simulink model "A1_PaceMaker"  (R2022a)
settings: Solver=FixedStepAuto  StartTime=0.0  StopTime=10.0  FixedStep=1e-3  RelTol=1e-3  EnableMultiTasking=on
undefined symbols (not defined in the file): D0, D1, D10, D11, D12, D13, D2, D3, D4, D5, D6, D7, D8, D9, PTA0, PTA1, PTA2, PTB23, PTB9, PTC16, PTC17, PTC2, PTC3, PTC4, PTD0, PTD1, PTD2, PTD3
libraries: frdmk64flib x14
settings Model: ExtModeTrigDuration=5  Creator=ramu7  LastModifiedBy=scoob
settings OptimizationCC: EnhancedBackFolding=on  PassReuseOutputArgsAs=Individual arguments  ZeroExternalMemoryAtStartup=off  ZeroInternalMemoryAtStartup=off  MaxStackSize=64  OptimizeBlockOrder=speed  DifferentSizesBufferReuse=on  OptimizationCustomize=off  EfficientTunableParamExpr=on
settings DebuggingCC: ParameterTunabilityLossMsg=error
settings HardwareCC: ProdBitPerPointer=32  ProdBitPerSizeT=32  ProdBitPerPtrDiffT=32  ProdLargestAtomicInteger=Long  ProdLargestAtomicFloat=Double  ProdWordSize=32  ProdHWDeviceType=ARM Compatible->ARM Cortex
settings SFSimCC: MATLABDynamicMemAlloc=off
settings RTWCC: SystemTargetFile=ert.tlc  HardwareBoard=NXP FRDM-K64F  TLCOptions="-aInlineSetEventsForThisBaseRateFcn=TLC_FALSE -aSuppressMultiTaskScheduler=TLC_FALSE  -aRateBasedStepFcn=0"  TemplateMakefile=ert_default_tmf  Toolchain=GNU Tools for ARM Embedded Processors
settings CodeAppCC: ForceParamTrailComments=on  IgnoreCustomStorageClasses=off  OperatorAnnotations=on  SimulinkDataObjDesc=on  SFDataObjDesc=on  InsertBlockDesc=on
settings ERTTargetCC: ExtModeTransport=4  ExtModeMexFile=sendToCommService

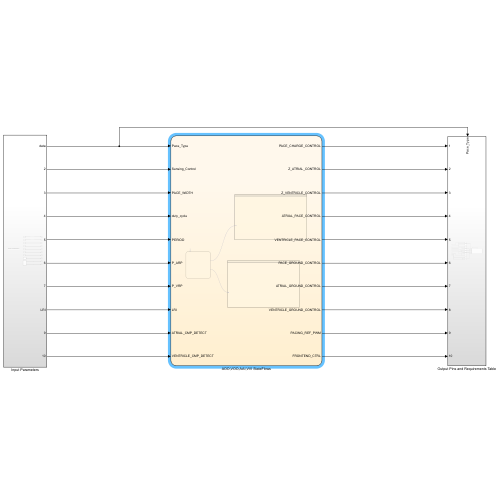
[thumbnail: Simulink's stored preview of the top-level diagram]
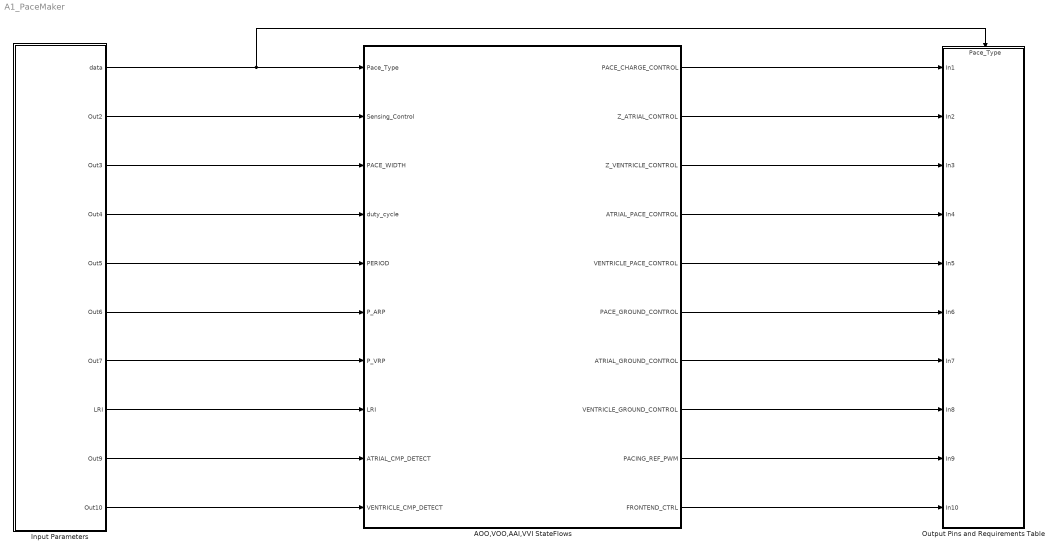
== system A1_PaceMaker ==
  AOO,VOO,AAI,VVI StateFlows : Stateflow chart  TreatAsAtomicUnit=on
      settings: PortSchema="{\"entries\":[{\"content\":{\"sides\":[{\"content\":{\"connectorIds\":[\"In2\",\"In10\",\"In7\",\"In1\",\"In3\",\"In9\",\"In8\",\"In6\",\"In4\",\"In5\"]},\"type\":\"ConnectorPlacement.EquallySpacedRectSide\",\"uuid\":\"9770646f-499d-4715-b3e0-54ec63e9a743\"},{\"content\":{\"connectorIds\":[\"Out1\",\"Out2\",\"Out3\",\"Out4\",\"Out5\",\"Out6\",\"Out7\",\"Out8\",\"Out9\",\"Out10\"],\"side\":\"RIGHT\"},\"type\":\"ConnectorPlacement.EquallySpacedRectSide\",\"uuid\":\"05a40026-c63e-4ef0-b71d-820a20f884f3\"},{\"content\":{\"connectorIds\":[],\"side\":\"TOP\"},\"type\":\"ConnectorPlacement.EquallySpacedRectSide\",\"uuid\":\"87d8712c-6353-4ad8-9661-243ca412d6bb\"}]},\"type\":\"ConnectorPlacement.EquallySpacedConnector\",\"uuid\":\"8262e7ac-98b5-44bf-add5-1ad3a0c707a1\"}],\"packageUris\":[\"http://schema.mathworks.com/mf0/Connector/R2020b\"],\"version\":\"1.0\"}"
  Input Parameters : Subsystem
  Output Pins and Requirements Table : Subsystem
      settings: PortSchema="{\"entries\":[{\"content\":{\"sides\":[{\"content\":{\"connectorIds\":[\"In1\",\"In2\",\"In3\",\"In4\",\"In5\",\"In6\",\"In7\",\"In8\",\"In9\",\"In10\"]},\"type\":\"ConnectorPlacement.EquallySpacedRectSide\",\"uuid\":\"40db26f6-8e31-4589-a315-6eea3b6d58f2\"},{\"content\":{\"connectorIds\":[],\"side\":\"RIGHT\"},\"type\":\"ConnectorPlacement.EquallySpacedRectSide\",\"uuid\":\"a6caef76-430e-44a7-94fa-313885a27199\"},{\"content\":{\"connectorIds\":[\"In11\"],\"side\":\"TOP\"},\"type\":\"ConnectorPlacement.EquallySpacedRectSide\",\"uuid\":\"9adbd5f8-a295-4590-a052-0a7aa200e456\"}]},\"type\":\"ConnectorPlacement.EquallySpacedConnector\",\"uuid\":\"6d560563-586d-4d61-8602-6a07324ae70c\"}],\"packageUris\":[\"http://schema.mathworks.com/mf0/Connector/R2020b\"],\"version\":\"1.0\"}"
  wires:
  AOO,VOO,AAI,VVI StateFlows/10(FRONTEND_CTRL) -> Output Pins and Requirements Table/10(In10)
  Input Parameters/8(LRI) -> AOO,VOO,AAI,VVI StateFlows/6(LRI)
  AOO,VOO,AAI,VVI StateFlows/6(PACE_GROUND_CONTROL) -> Output Pins and Requirements Table/6(In6)
  AOO,VOO,AAI,VVI StateFlows/2(Z_ATRIAL_CONTROL) -> Output Pins and Requirements Table/2(In2)
  AOO,VOO,AAI,VVI StateFlows/3(Z_VENTRICLE_CONTROL) -> Output Pins and Requirements Table/3(In3)
  AOO,VOO,AAI,VVI StateFlows/1(PACE_CHARGE_CONTROL) -> Output Pins and Requirements Table/1(In1)
  AOO,VOO,AAI,VVI StateFlows/4(ATRIAL_PACE_CONTROL) -> Output Pins and Requirements Table/4(In4)
  Input Parameters/3(Out3) -> AOO,VOO,AAI,VVI StateFlows/7(PACE_WIDTH)
  AOO,VOO,AAI,VVI StateFlows/9(PACING_REF_PWM) -> Output Pins and Requirements Table/9(In9)
  Input Parameters/2(Out2) -> AOO,VOO,AAI,VVI StateFlows/10(Sensing_Control)
  Input Parameters/5(Out5) -> AOO,VOO,AAI,VVI StateFlows/3(PERIOD)
  AOO,VOO,AAI,VVI StateFlows/7(ATRIAL_GROUND_CONTROL) -> Output Pins and Requirements Table/7(In7)
  Input Parameters/9(Out9) -> AOO,VOO,AAI,VVI StateFlows/4(ATRIAL_CMP_DETECT)
  Input Parameters/4(Out4) -> AOO,VOO,AAI,VVI StateFlows/1(duty_cycle)
  AOO,VOO,AAI,VVI StateFlows/5(VENTRICLE_PACE_CONTROL) -> Output Pins and Requirements Table/5(In5)
  Input Parameters/7(Out7) -> AOO,VOO,AAI,VVI StateFlows/8(P_VRP)
  Input Parameters/10(Out10) -> AOO,VOO,AAI,VVI StateFlows/5(VENTRICLE_CMP_DETECT)
  AOO,VOO,AAI,VVI StateFlows/8(VENTRICLE_GROUND_CONTROL) -> Output Pins and Requirements Table/8(In8)
  Input Parameters/6(Out6) -> AOO,VOO,AAI,VVI StateFlows/9(P_ARP)
  Input Parameters/1(data) -> Output Pins and Requirements Table/11(Pace_Type), AOO,VOO,AAI,VVI StateFlows/2(Pace_Type)

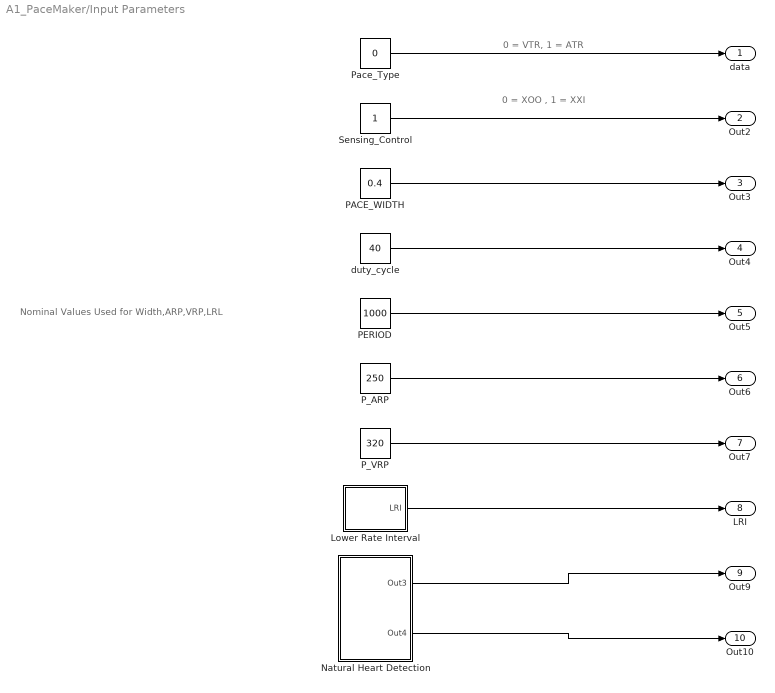
== system A1_PaceMaker/Input Parameters ==
  note: Nominal Values Used for Width,ARP,VRP,LRL
  note: 0 = XOO , 1 = XXI
  note: 0 = VTR, 1 = ATR
  Lower Rate Interval : Subsystem
  Natural Heart Detection : Subsystem
  PACE_WIDTH : Constant  Value=0.4
  PERIOD : Constant  Value=1000
  P_ARP : Constant  Value=250
  P_VRP : Constant  Value=320
  Pace_Type : Constant  Value=0  OutDataTypeStr=boolean
  Sensing_Control : Constant  OutDataTypeStr=boolean
  duty_cycle : Constant  Value=40  OutDataTypeStr=double
  data : Outport
  Out2 : Outport  Port=2
  Out3 : Outport  Port=3
  Out4 : Outport  Port=4
  Out5 : Outport  Port=5
  Out6 : Outport  Port=6
  Out7 : Outport  Port=7
  LRI : Outport  Port=8
  Out9 : Outport  Port=9
  Out10 : Outport  Port=10
  wires:
  Lower Rate Interval/1(LRI) -> LRI/1
  PERIOD/1 -> Out5/1
  P_VRP/1 -> Out7/1
  duty_cycle/1 -> Out4/1
  Sensing_Control/1 -> Out2/1
  PACE_WIDTH/1 -> Out3/1
  Natural Heart Detection/2(Out4) -> Out10/1
  P_ARP/1 -> Out6/1
  Pace_Type/1 -> data/1
  Natural Heart Detection/1(Out3) -> Out9/1

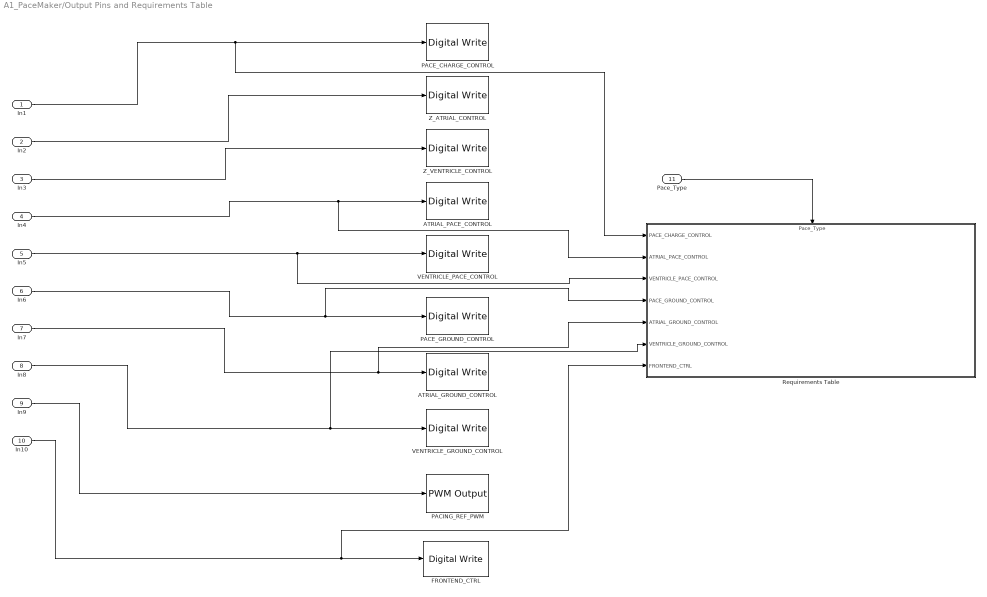
== system A1_PaceMaker/Output Pins and Requirements Table ==
  In1 : Inport
  In2 : Inport  Port=2
  In3 : Inport  Port=3
  In4 : Inport  Port=4
  In5 : Inport  Port=5
  In6 : Inport  Port=6
  In7 : Inport  Port=7
  In8 : Inport  Port=8
  In9 : Inport  Port=9
  In10 : Inport  Port=10
  Pace_Type : Inport  Port=11
  ATRIAL_GROUND_CONTROL : frdmk64flib/Digital Write  Whichpin=PTD2 (D11)
  ATRIAL_PACE_CONTROL : frdmk64flib/Digital Write  Whichpin=PTA0 (D8)
  FRONTEND_CTRL : frdmk64flib/Digital Write  Whichpin=PTD1 (D13)
  PACE_CHARGE_CONTROL : frdmk64flib/Digital Write  Whichpin=PTB9 (D2)
  PACE_GROUND_CONTROL : frdmk64flib/Digital Write  Whichpin=PTD0 (D10)
  PACING_REF_PWM : frdmk64flib/PWM Output  Whichpin=PTA2 (D5)  InitialFrequency=2000  InitialDutyCycle=40
  Requirements Table : Subsystem
      settings: PortSchema="{\"entries\":[{\"content\":{\"sides\":[{\"content\":{\"connectorIds\":[\"In1\",\"In2\",\"In3\",\"In4\",\"In5\",\"In6\",\"In7\"]},\"type\":\"ConnectorPlacement.EquallySpacedRectSide\",\"uuid\":\"46327938-4478-40d2-aac6-72547228615e\"},{\"content\":{\"connectorIds\":[],\"side\":\"RIGHT\"},\"type\":\"ConnectorPlacement.EquallySpacedRectSide\",\"uuid\":\"a4c12f67-beb4-4537-be9d-262931108289\"},{\"content\":{\"connectorIds\":[\"In8\"],\"side\":\"TOP\"},\"type\":\"ConnectorPlacement.EquallySpacedRectSide\",\"uuid\":\"a653f2ff-3266-45dd-85b5-df796fc313fd\"}]},\"type\":\"ConnectorPlacement.EquallySpacedConnector\",\"uuid\":\"ede91063-bb98-4867-a1df-25b64c24a60e\"}],\"packageUris\":[\"http://schema.mathworks.com/mf0/Connector/R2020b\"],\"version\":\"1.0\"}"
  VENTRICLE_GROUND_CONTROL : frdmk64flib/Digital Write  Whichpin=PTD3 (D12)
  VENTRICLE_PACE_CONTROL : frdmk64flib/Digital Write  Whichpin=PTC4 (D9)
  Z_ATRIAL_CONTROL : frdmk64flib/Digital Write  Whichpin=PTB23 (D4)
  Z_VENTRICLE_CONTROL : frdmk64flib/Digital Write  Whichpin=PTC3 (D7)
  wires:
  In2/1 -> Z_ATRIAL_CONTROL/1
  In9/1 -> PACING_REF_PWM/1
  In5/1 -> Requirements Table/3(VENTRICLE_PACE_CONTROL), VENTRICLE_PACE_CONTROL/1
  In7/1 -> Requirements Table/5(ATRIAL_GROUND_CONTROL), ATRIAL_GROUND_CONTROL/1
  In4/1 -> Requirements Table/2(ATRIAL_PACE_CONTROL), ATRIAL_PACE_CONTROL/1
  In8/1 -> Requirements Table/6(VENTRICLE_GROUND_CONTROL), VENTRICLE_GROUND_CONTROL/1
  In6/1 -> Requirements Table/4(PACE_GROUND_CONTROL), PACE_GROUND_CONTROL/1
  In1/1 -> Requirements Table/1(PACE_CHARGE_CONTROL), PACE_CHARGE_CONTROL/1
  In3/1 -> Z_VENTRICLE_CONTROL/1
  In10/1 -> Requirements Table/7(FRONTEND_CTRL), FRONTEND_CTRL/1
  Pace_Type/1 -> Requirements Table/8(Pace_Type)

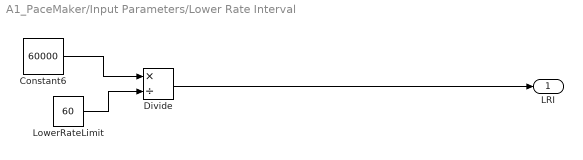
== system A1_PaceMaker/Input Parameters/Lower Rate Interval ==
  Constant6 : Constant  Value=60000
  Divide : Product  Inputs=*/
  LowerRateLimit : Constant  Value=60
  LRI : Outport
  wires:
  Constant6/1 -> Divide/1
  LowerRateLimit/1 -> Divide/2
  Divide/1 -> LRI/1

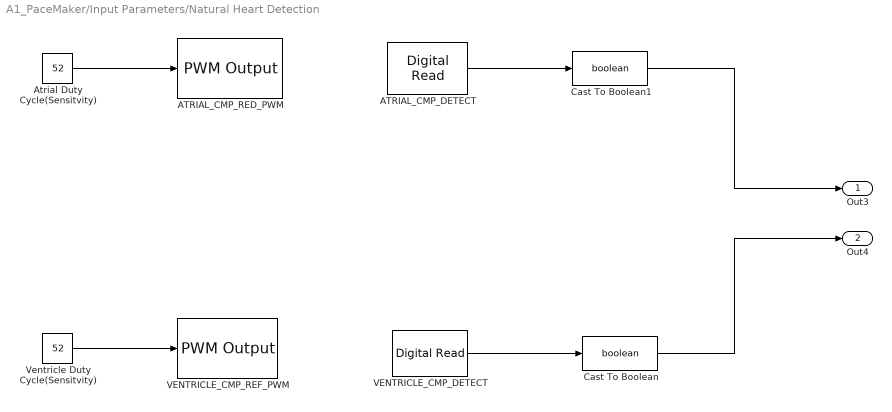
== system A1_PaceMaker/Input Parameters/Natural Heart Detection ==
  ATRIAL_CMP_DETECT : frdmk64flib/Digital Read  Whichpin=PTC16 (D0)  SampleTime=-1
  ATRIAL_CMP_RED_PWM : frdmk64flib/PWM Output  Whichpin=PTC2 (D6)  InitialFrequency=2000  InitialDutyCycle=51
  Atrial Duty Cycle(Sensitvity) : Constant  Value=52
  Cast To Boolean : DataTypeConversion  OutDataTypeStr=boolean  SaturateOnIntegerOverflow=off  RndMeth=Floor
  Cast To Boolean1 : DataTypeConversion  OutDataTypeStr=boolean  SaturateOnIntegerOverflow=off  RndMeth=Floor
  VENTRICLE_CMP_DETECT : frdmk64flib/Digital Read  Whichpin=PTC17 (D1)  SampleTime=-1
  VENTRICLE_CMP_REF_PWM : frdmk64flib/PWM Output  Whichpin=PTA1 (D3)  InitialFrequency=2000  InitialDutyCycle=60
  Ventricle Duty Cycle(Sensitvity) : Constant  Value=52
  Out3 : Outport
  Out4 : Outport  Port=2
  wires:
  Ventricle Duty Cycle(Sensitvity)/1 -> VENTRICLE_CMP_REF_PWM/1
  Atrial Duty Cycle(Sensitvity)/1 -> ATRIAL_CMP_RED_PWM/1
  VENTRICLE_CMP_DETECT/1 -> Cast To Boolean/1
  ATRIAL_CMP_DETECT/1 -> Cast To Boolean1/1
  Cast To Boolean1/1 -> Out3/1
  Cast To Boolean/1 -> Out4/1

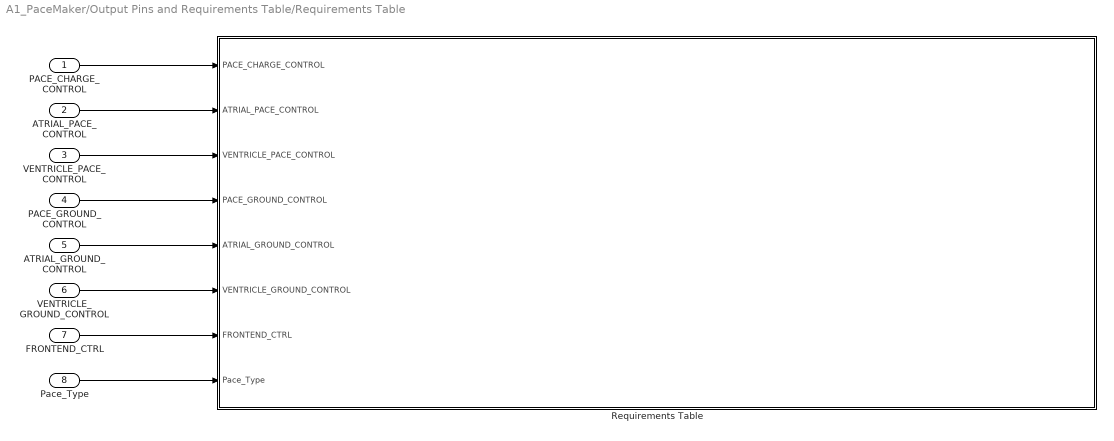
== system A1_PaceMaker/Output Pins and Requirements Table/Requirements Table ==
  PACE_CHARGE_CONTROL : Inport
  ATRIAL_PACE_CONTROL : Inport  Port=2
  VENTRICLE_PACE_CONTROL : Inport  Port=3
  PACE_GROUND_CONTROL : Inport  Port=4
  ATRIAL_GROUND_CONTROL : Inport  Port=5
  VENTRICLE_GROUND_CONTROL : Inport  Port=6
  FRONTEND_CTRL : Inport  Port=7
  Pace_Type : Inport  Port=8
  Requirements Table : Requirements Table  TreatAsAtomicUnit=on
  wires:
  PACE_CHARGE_CONTROL/1 -> Requirements Table/1(PACE_CHARGE_CONTROL)
  ATRIAL_PACE_CONTROL/1 -> Requirements Table/2(ATRIAL_PACE_CONTROL)
  VENTRICLE_PACE_CONTROL/1 -> Requirements Table/3(VENTRICLE_PACE_CONTROL)
  PACE_GROUND_CONTROL/1 -> Requirements Table/4(PACE_GROUND_CONTROL)
  ATRIAL_GROUND_CONTROL/1 -> Requirements Table/5(ATRIAL_GROUND_CONTROL)
  VENTRICLE_GROUND_CONTROL/1 -> Requirements Table/6(VENTRICLE_GROUND_CONTROL)
  FRONTEND_CTRL/1 -> Requirements Table/7(FRONTEND_CTRL)
  Pace_Type/1 -> Requirements Table/8(Pace_Type)

== stateflow chart A1_PaceMaker/AOO,VOO,AAI,VVI StateFlows ==
  state VENTRICLE MODES (VOO and VVI) [group]
    state SENSE_Ventricle
    note: Heartbeat not found after the LRI period, pace the heart
    note: Heartbeat found, reset LRI
    state PACE_Charge_Ventricle
      entry:
      PACE_CHARGE_CONTROL = true
      VENTRICLE_PACE_CONTROL = false
      VENTRICLE_GROUND_CONTROL=true
      ATRIAL_PACE_CONTROL =false
      ATRIAL_GROUND_CONTROL = false
    state PACE_Discharge_Ventricle
      entry:
      PACE_CHARGE_CONTROL = false
      VENTRICLE_PACE_CONTROL = true
      VENTRICLE_GROUND_CONTROL= false
    SENSE_Ventricle -> PACE_Discharge_Ventricle [order 1] : after(LRI - P_VRP,msec) [VENTRICLE_CMP_DETECT == false]
    SENSE_Ventricle -> PACE_Charge_Ventricle [order 2] : [VENTRICLE_CMP_DETECT == true]
    PACE_Charge_Ventricle -> SENSE_Ventricle [order 1] : after(P_VRP,msec)[Sensing_Control == true]
    PACE_Charge_Ventricle -> PACE_Discharge_Ventricle [order 2] : after(PERIOD - PACE_WIDTH,msec)[Sensing_Control == false]
    PACE_Discharge_Ventricle -> PACE_Charge_Ventricle : after(PACE_WIDTH,msec)
  state init_state
    entry:
    PACING_REF_PWM = duty_cycle
    Z_ATRIAL_CONTROL = false
    Z_VENTRICLE_CONTROL = false
    PACE_GROUND_CONTROL = true
    FRONTEND_CTRL = true
  state ATRIAL MODES (AOO and AAI) [group]
    state SENSE_Atrial
    note: Heartbeat not found after the LRI period, pace the heart
    note: Heartbeat found, reset LRI
    state PACE_Charge_Atrial
      entry:
      PACE_CHARGE_CONTROL = true
      VENTRICLE_PACE_CONTROL = false
      VENTRICLE_GROUND_CONTROL=false
      ATRIAL_PACE_CONTROL =false
      ATRIAL_GROUND_CONTROL = true
    state PACE_Discharge_Atrial
      entry:
      PACE_CHARGE_CONTROL = false
      ATRIAL_PACE_CONTROL = true
      ATRIAL_GROUND_CONTROL = false
    SENSE_Atrial -> PACE_Discharge_Atrial [order 1] : after(LRI - P_ARP - PACE_WIDTH,msec) [ATRIAL_CMP_DETECT == false]
    SENSE_Atrial -> PACE_Charge_Atrial [order 2] : [ATRIAL_CMP_DETECT == true]
    PACE_Charge_Atrial -> SENSE_Atrial [order 1] : after(P_ARP,msec) [Sensing_Control == true]
    PACE_Charge_Atrial -> PACE_Discharge_Atrial [order 2] : after(PERIOD - PACE_WIDTH,msec)[Sensing_Control == false]
    PACE_Discharge_Atrial -> PACE_Charge_Atrial : after(PACE_WIDTH,msec)
  init_state -> PACE_Charge_Ventricle [order 2] : [Pace_Type == 0]
  (default) -> init_state
  init_state -> PACE_Charge_Atrial [order 1] : [Pace_Type == 1]
  data: PACE_CHARGE_CONTROL output; Z_ATRIAL_CONTROL output; Z_VENTRICLE_CONTROL output; ATRIAL_PACE_CONTROL output; VENTRICLE_PACE_CONTROL output; PACE_GROUND_CONTROL output; ATRIAL_GROUND_CONTROL output; VENTRICLE_GROUND_CONTROL output; PACING_REF_PWM output; duty_cycle input; Pace_Type input boolean; PERIOD input double; ATRIAL_CMP_DETECT input boolean; VENTRICLE_CMP_DETECT input boolean; LRI input double; PACE_WIDTH input double; P_VRP input double; P_ARP input double; Sensing_Control input boolean; FRONTEND_CTRL output boolean

== stateflow chart A1_PaceMaker/Output Pins and Requirements Table/Requirements Table/Requirements Table ==
  (default) -> (junction 1073754047)
  (junction 1073754047) -> (junction 1073754048) : {
      | % SF_REQ_REV_07
      | }
  (junction 1073754048) -> (junction 1073754050) : {
      | % HEADER_ASSIGNMENTS
      |
      | }
  (junction 1073754050) -> (junction 1073754052) : {
      | % START_A_4
      | }
  (junction 1073754052) -> (junction 1073754054) : {
      | }
  (junction 1073754054) -> (junction 1073754056)
  (junction 1073754056) -> (junction 1073754058) : {
      | }
  (junction 1073754058) -> (junction 1073754060) : {
      | % END_A_4
      | }
  (junction 1073754060) -> (junction 1073754062) : {
      | % START_R_1
      | }
  (junction 1073754062) -> (junction 1073754064) : {
      | }
  (junction 1073754064) -> (junction 1073754066)
  (junction 1073754066) -> (junction 1073754068) [order 1] : [(((Front End Control) == (FRONTEND_CTRL==1))) && (((Pace Ground Control) == (PACE_GROUND_CONTROL==1))) && (((Z Atrial Control) == (Z_ATRIAL_CONTROL==0))) && (((Z Ventricular Control) == (Z_VENTRICLE_CONTROL==0))) && (((Pace Type) == (Pace_Type==1)))]
  (junction 1073754066) -> (junction 1073754164) [order 2]
  (junction 1073754068) -> (junction 1073754070) : {
      | reqtable_postcondition((((PACE_CHARGE_CONTROL) == (1))) && (((VENTRICLE_PACE_CONTROL) == (0))) && (((VENTRICLE_GROUND_CONTROL) == (0))) && (((ATRIAL_PACE_CONTROL) == (0))) && (((ATRIAL_GROUND_CONTROL) == (1))), 'R:1');
      |
      |
      | }
  (junction 1073754070) -> (junction 1073754072) : {
      | }
  (junction 1073754072) -> (junction 1073754074) : {
      | % START_R_10
      | }
  (junction 1073754074) -> (junction 1073754076) : {
      | }
  (junction 1073754076) -> (junction 1073754078)
  (junction 1073754078) -> (junction 1073754080) [order 1] : [(((Pace Charge Control) == (PACE_CHARGE_CONTROL==1))) && (((Ventricle Pace Control) == (VENTRICLE_PACE_CONTROL==0))) && (((Ventricle Ground Control) == (VENTRICLE_GROUND_CONTROL==0))) && (((Atrial Pace Control) == (ATRIAL_PACE_CONTROL==0))) && (((Atrial Ground Control) == (ATRIAL_GROUND_CONTROL==1))) && (((Sensing Control) == (Sensing_Control==0)))]
  (junction 1073754078) -> (junction 1073754086) [order 2]
  (junction 1073754080) -> (junction 1073754082) : {
      | reqtable_postcondition((((PACE_CHARGE_CONTROL) == (0))) && (((ATRIAL_PACE_CONTROL) == (1))) && (((ATRIAL_GROUND_CONTROL) == (0))), 'R:1.1');
      |
      |
      | }
  (junction 1073754082) -> (junction 1073754084) : {
      | }
  (junction 1073754084) -> (junction 1073754086)
  (junction 1073754086) -> (junction 1073754088)
  (junction 1073754088) -> (junction 1073754090) : {
      | % END_R_10
      | }
  (junction 1073754090) -> (junction 1073754092) : {
      | % START_R_16
      | }
  (junction 1073754092) -> (junction 1073754094) : {
      | }
  (junction 1073754094) -> (junction 1073754096)
  (junction 1073754096) -> (junction 1073754098) [order 1] : [(((Pace Charge Control) == (PACE_CHARGE_CONTROL==0))) && (((Atrial Pace Control) == (ATRIAL_PACE_CONTROL==1))) && (((Atrial Ground Control) == (ATRIAL_GROUND_CONTROL==0)))]
  (junction 1073754096) -> (junction 1073754104) [order 2]
  (junction 1073754098) -> (junction 1073754100) : {
      | reqtable_postcondition((((PACE_CHARGE_CONTROL) == (1))) && (((VENTRICLE_PACE_CONTROL) == (0))) && (((VENTRICLE_GROUND_CONTROL) == (0))) && (((ATRIAL_PACE_CONTROL) == (0))) && (((ATRIAL_GROUND_CONTROL) == (1))), 'R:1.2');
      |
      |
      | }
  (junction 1073754100) -> (junction 1073754102) : {
      | }
  (junction 1073754102) -> (junction 1073754104)
  (junction 1073754104) -> (junction 1073754106)
  (junction 1073754106) -> (junction 1073754108) : {
      | % END_R_16
      | }
  (junction 1073754108) -> (junction 1073754110) : {
      | % START_R_19
      | }
  (junction 1073754110) -> (junction 1073754112) : {
      | }
  (junction 1073754112) -> (junction 1073754114)
  (junction 1073754114) -> (junction 1073754116) [order 1] : [(((Pace Charge Control) == (PACE_CHARGE_CONTROL==1))) && (((Ventricle Pace Control) == (VENTRICLE_PACE_CONTROL==0))) && (((Ventricle Ground Control) == (VENTRICLE_GROUND_CONTROL==0))) && (((Atrial Pace Control) == (ATRIAL_PACE_CONTROL==0))) && (((Atrial Ground Control) == (ATRIAL_GROUND_CONTROL==1))) && (((Sensing Control) == (Sensing_Control==1)))]
  (junction 1073754114) -> (junction 1073754122) [order 2]
  (junction 1073754116) -> (junction 1073754118) : {
      |
      |
      | }
  (junction 1073754118) -> (junction 1073754120) : {
      | }
  (junction 1073754120) -> (junction 1073754122)
  (junction 1073754122) -> (junction 1073754124)
  (junction 1073754124) -> (junction 1073754126) : {
      | % END_R_19
      | }
  (junction 1073754126) -> (junction 1073754128) : {
      | % START_R_28
      | }
  (junction 1073754128) -> (junction 1073754130) : {
      | }
  (junction 1073754130) -> (junction 1073754132)
  (junction 1073754132) -> (junction 1073754134) [order 1] : [(((Atrial CMP Detect) == (ATRIAL_CMP_DETECT==1)))]
  (junction 1073754132) -> (junction 1073754140) [order 2]
  (junction 1073754134) -> (junction 1073754136) : {
      | reqtable_postcondition((((PACE_CHARGE_CONTROL) == (1))) && (((VENTRICLE_PACE_CONTROL) == (0))) && (((VENTRICLE_GROUND_CONTROL) == (0))) && (((ATRIAL_PACE_CONTROL) == (0))) && (((ATRIAL_GROUND_CONTROL) == (1))), 'R:1.4');
      |
      |
      | }
  (junction 1073754136) -> (junction 1073754138) : {
      | }
  (junction 1073754138) -> (junction 1073754140)
  (junction 1073754140) -> (junction 1073754142)
  (junction 1073754142) -> (junction 1073754144) : {
      | % END_R_28
      | }
  (junction 1073754144) -> (junction 1073754146) : {
      | % START_R_31
      | }
  (junction 1073754146) -> (junction 1073754148) : {
      | }
  (junction 1073754148) -> (junction 1073754150)
  (junction 1073754150) -> (junction 1073754152) [order 1] : [(((Atrial CMP Detect) == (ATRIAL_CMP_DETECT==0)))]
  (junction 1073754150) -> (junction 1073754158) [order 2]
  (junction 1073754152) -> (junction 1073754154) : {
      | reqtable_postcondition((((PACE_CHARGE_CONTROL) == (0))) && (((ATRIAL_PACE_CONTROL) == (1))) && (((ATRIAL_GROUND_CONTROL) == (0))), 'R:1.5');
      |
      |
      | }
  (junction 1073754154) -> (junction 1073754156) : {
      | }
  (junction 1073754156) -> (junction 1073754158)
  (junction 1073754158) -> (junction 1073754160)
  (junction 1073754160) -> (junction 1073754162) : {
      | % END_R_31
      | }
  (junction 1073754162) -> (junction 1073754164)
  (junction 1073754164) -> (junction 1073754166)
  (junction 1073754166) -> (junction 1073754168) : {
      | % END_R_1
      | }
  (junction 1073754168) -> (junction 1073754170) : {
      | % START_R_7
      | }
  (junction 1073754170) -> (junction 1073754172) : {
      | }
  (junction 1073754172) -> (junction 1073754174)
  (junction 1073754174) -> (junction 1073754176) [order 1] : [(((Front End Control) == (FRONTEND_CTRL==1))) && (((Pace Ground Control) == (PACE_GROUND_CONTROL==1))) && (((Z Atrial Control) == (Z_ATRIAL_CONTROL==0))) && (((Z Ventricular Control) == (Z_VENTRICLE_CONTROL==0))) && (((Pace Type) == (Pace_Type==0)))]
  (junction 1073754174) -> (junction 1073754272) [order 2]
  (junction 1073754176) -> (junction 1073754178) : {
      | reqtable_postcondition((((PACE_CHARGE_CONTROL) == (1))) && (((VENTRICLE_PACE_CONTROL) == (0))) && (((VENTRICLE_GROUND_CONTROL) == (1))) && (((ATRIAL_PACE_CONTROL) == (0))) && (((ATRIAL_GROUND_CONTROL) == (0))), 'R:2');
      |
      |
      | }
  (junction 1073754178) -> (junction 1073754180) : {
      | }
  (junction 1073754180) -> (junction 1073754182) : {
      | % START_R_13
      | }
  (junction 1073754182) -> (junction 1073754184) : {
      | }
  (junction 1073754184) -> (junction 1073754186)
  (junction 1073754186) -> (junction 1073754188) [order 1] : [(((Pace Charge Control) == (PACE_CHARGE_CONTROL==1))) && (((Ventricle Pace Control) == (VENTRICLE_PACE_CONTROL==0))) && (((Ventricle Ground Control) == (VENTRICLE_GROUND_CONTROL==1))) && (((Atrial Pace Control) == (ATRIAL_PACE_CONTROL==0))) && (((Atrial Ground Control) == (ATRIAL_GROUND_CONTROL==0))) && (((Sensing Control) == (Sensing_Control==0)))]
  (junction 1073754186) -> (junction 1073754194) [order 2]
  (junction 1073754188) -> (junction 1073754190) : {
      | reqtable_postcondition((((PACE_CHARGE_CONTROL) == (0))) && (((VENTRICLE_PACE_CONTROL) == (1))) && (((VENTRICLE_GROUND_CONTROL) == (0))), 'R:2.1');
      |
      |
      | }
  (junction 1073754190) -> (junction 1073754192) : {
      | }
  (junction 1073754192) -> (junction 1073754194)
  (junction 1073754194) -> (junction 1073754196)
  (junction 1073754196) -> (junction 1073754198) : {
      | % END_R_13
      | }
  (junction 1073754198) -> (junction 1073754200) : {
      | % START_R_22
      | }
  (junction 1073754200) -> (junction 1073754202) : {
      | }
  (junction 1073754202) -> (junction 1073754204)
  (junction 1073754204) -> (junction 1073754206) [order 1] : [(((Pace Charge Control) == (PACE_CHARGE_CONTROL==0))) && (((Ventricle Pace Control) == (VENTRICLE_PACE_CONTROL==1))) && (((Ventricle Ground Control) == (VENTRICLE_GROUND_CONTROL==0)))]
  (junction 1073754204) -> (junction 1073754212) [order 2]
  (junction 1073754206) -> (junction 1073754208) : {
      | reqtable_postcondition((((PACE_CHARGE_CONTROL) == (1))) && (((VENTRICLE_PACE_CONTROL) == (0))) && (((VENTRICLE_GROUND_CONTROL) == (1))) && (((ATRIAL_PACE_CONTROL) == (0))) && (((ATRIAL_GROUND_CONTROL) == (0))), 'R:2.2');
      |
      |
      | }
  (junction 1073754208) -> (junction 1073754210) : {
      | }
  (junction 1073754210) -> (junction 1073754212)
  (junction 1073754212) -> (junction 1073754214)
  (junction 1073754214) -> (junction 1073754216) : {
      | % END_R_22
      | }
  (junction 1073754216) -> (junction 1073754218) : {
      | % START_R_25
      | }
  (junction 1073754218) -> (junction 1073754220) : {
      | }
  (junction 1073754220) -> (junction 1073754222)
  (junction 1073754222) -> (junction 1073754224) [order 1] : [(((Pace Charge Control) == (PACE_CHARGE_CONTROL==1))) && (((Ventricle Pace Control) == (VENTRICLE_PACE_CONTROL==0))) && (((Ventricle Ground Control) == (VENTRICLE_GROUND_CONTROL==1))) && (((Atrial Pace Control) == (ATRIAL_PACE_CONTROL==0))) && (((Atrial Ground Control) == (ATRIAL_GROUND_CONTROL==0))) && (((Sensing Control) == (Sensing_Control==1)))]
  (junction 1073754222) -> (junction 1073754230) [order 2]
  (junction 1073754224) -> (junction 1073754226) : {
      |
      |
      | }
  (junction 1073754226) -> (junction 1073754228) : {
      | }
  (junction 1073754228) -> (junction 1073754230)
  (junction 1073754230) -> (junction 1073754232)
  (junction 1073754232) -> (junction 1073754234) : {
      | % END_R_25
      | }
  (junction 1073754234) -> (junction 1073754236) : {
      | % START_R_34
      | }
  (junction 1073754236) -> (junction 1073754238) : {
      | }
  (junction 1073754238) -> (junction 1073754240)
  (junction 1073754240) -> (junction 1073754242) [order 1] : [(((Ventricle CMP Detect) == (VENTRICLE_CMP_DETECT==1)))]
  (junction 1073754240) -> (junction 1073754248) [order 2]
  (junction 1073754242) -> (junction 1073754244) : {
      | reqtable_postcondition((((PACE_CHARGE_CONTROL) == (1))) && (((VENTRICLE_PACE_CONTROL) == (0))) && (((VENTRICLE_GROUND_CONTROL) == (1))) && (((ATRIAL_PACE_CONTROL) == (0))) && (((ATRIAL_GROUND_CONTROL) == (0))), 'R:2.4');
      |
      |
      | }
  (junction 1073754244) -> (junction 1073754246) : {
      | }
  (junction 1073754246) -> (junction 1073754248)
  (junction 1073754248) -> (junction 1073754250)
  (junction 1073754250) -> (junction 1073754252) : {
      | % END_R_34
      | }
  (junction 1073754252) -> (junction 1073754254) : {
      | % START_R_37
      | }
  (junction 1073754254) -> (junction 1073754256) : {
      | }
  (junction 1073754256) -> (junction 1073754258)
  (junction 1073754258) -> (junction 1073754260) [order 1] : [(((Ventricle CMP Detect) == (VENTRICLE_CMP_DETECT==1)))]
  (junction 1073754258) -> (junction 1073754266) [order 2]
  (junction 1073754260) -> (junction 1073754262) : {
      | reqtable_postcondition((((PACE_CHARGE_CONTROL) == (0))) && (((VENTRICLE_PACE_CONTROL) == (1))) && (((VENTRICLE_GROUND_CONTROL) == (0))), 'R:2.5');
      |
      |
      | }
  (junction 1073754262) -> (junction 1073754264) : {
      | }
  (junction 1073754264) -> (junction 1073754266)
  (junction 1073754266) -> (junction 1073754268)
  (junction 1073754268) -> (junction 1073754270) : {
      | % END_R_37
      | }
  (junction 1073754270) -> (junction 1073754272)
  (junction 1073754272) -> (junction 1073754274)
  (junction 1073754274) -> (junction 1073754276) : {
      | % END_R_7
      | }
  data: PACE_CHARGE_CONTROL input boolean; ATRIAL_PACE_CONTROL input boolean; VENTRICLE_PACE_CONTROL input boolean; PACE_GROUND_CONTROL input boolean; ATRIAL_GROUND_CONTROL input boolean; VENTRICLE_GROUND_CONTROL input boolean; FRONTEND_CTRL input boolean; Pace_Type input boolean
